simulink model "ANFIS"  (R2015a)
settings: Solver=ode45  StartTime=0.02  StopTime=0.04  RelTol=1e-3
libraries: simulink x36, powerlib_meascontrol x30, powerlib x19, fuzblock x8
(part 1 of 2)
settings Model: Creator=Yahya  LastModifiedBy=Yahya

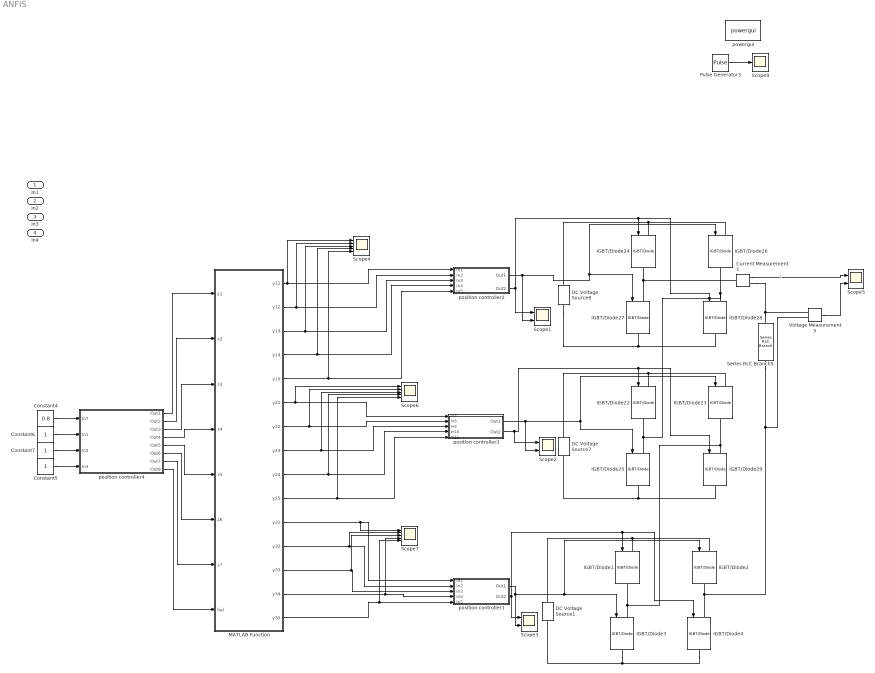
== system ANFIS ==
  note: i
  In1 : Inport
  In2 : Inport  Port=2
  In3 : Inport  Port=3
  In4 : Inport  Port=4
  Constant4 : Constant  Value=0.8
  Constant5 : Constant
  Constant6 : Constant
  Constant7 : Constant
  Current Measurement1 : powerlib/Measurements/Current Measurement  PhasorSimulation=off  OutputType=Complex  PSBequivalent=0
  DC Voltage Source1 : powerlib/Electrical Sources/DC Voltage Source  Amplitude=100  Measurements=None
  DC Voltage Source7 : powerlib/Electrical Sources/DC Voltage Source  Amplitude=100  Measurements=None
  DC Voltage Source8 : powerlib/Electrical Sources/DC Voltage Source  Amplitude=100  Measurements=None
  IGBT/Diode{1..4,22..29} (12 alike) : powerlib/Power Electronics/IGBT//Diode  Ron=1e-3  Rs=1e5  Cs=inf  Measurements=off
  MATLAB Function : MATLAB Function  TreatAsAtomicUnit=on
  Pulse Generator3 : DiscretePulseGenerator  PulseType=Time based  Amplitude=0.8  Period=0.00001  PulseWidth=50
  Scope{1..3,5} (4 alike) : Scope  NumInputPorts=2
      Scope1 settings: TimeRange=1  YMin=-400~-400  YMax=400~400  SaveName=ScopeData7
      Scope2 settings: TimeRange=1  YMin=-400~-400  YMax=400~400  SaveName=ScopeData8
      Scope3 settings: TimeRange=1  YMin=-400~-400  YMax=400~400  SaveName=ScopeData9
      Scope5 settings: TimeRange=1  YMin=-400~-400  YMax=400~400  SaveName=ScopeData3
  Scope4 : Scope  NumInputPorts=5
      settings: TimeRange=1  YMin=-400~-400~-5~-5~-5  YMax=400~400~5~5~5  SaveName=ScopeData12
  Scope6 : Scope  NumInputPorts=5
      settings: TimeRange=1  YMin=-400~-400~-5~-5~-5  YMax=400~400~5~5~5  SaveName=ScopeData13
  Scope7 : Scope  NumInputPorts=5
      settings: TimeRange=1  YMin=-400~-400~-5~-5~-5  YMax=400~400~5~5~5  SaveName=ScopeData14
  Scope9 : Scope
      settings: SaveName=ScopeData18
  Series RLC Branch5 : powerlib/Elements/Series RLC Branch  LConnTagsString=__new0  RConnTagsString=__new0  BranchType=R  Resistance=3000  Inductance=1e-5  SetiL0=off  InitialCurrent=0  Capacitance=1e-6  Setx0=off  InitialVoltage=0  Measurements=None
  Voltage Measurement5 : powerlib/Measurements/Voltage Measurement  PhasorSimulation=off  OutputType=Complex  PSBequivalent=0
  position controller1 : Subsystem
  position controller2 : Subsystem
  position controller3 : Subsystem
  position controller4 : Subsystem
  powergui : powerlib/powergui  Priority=1  SimulationMode=Continuous  SolverType=Tustin/Backward Euler (TBE)  SampleTime=50e-6  frequency=60  SPID=off  DisableSnubberDevices=off  DisableRonSwitches=off  DisableVfSwitches=off  SwTol=0  DisplayEquations=off  Interpol=off  methode=off  Ts=100  FunctionMessages=off  echomessages=off  HookPort=off  EnableUseOfTLC=off  x0status=blocks  frequencyindice=0  Pbase=100e6  ErrMax=1e-4  Iterations=50  UnitsV=kV  UnitsW=MW  buscounter=0  RestoreLinks=warning  ResistiveCurrentMeasurement=off  Frange=[0:2:500]  Ylog=off  Xlog=on  ShowGrid=off  save=off  variable=ZData  structure=0  ZoomFFT=off  StartTime=0.0  cycles=1  DisplayStyle=1  fundamental=60  FreqAxis=off  MaxFrequency=1000  frequencyindicesteady=1  RmsSteady=1  display=off
  wires:
  position controller2/2(Out2) -> Scope1/1, IGBT/Diode28/1, IGBT/Diode24/1
  position controller2/1(Out1) -> Scope1/2, IGBT/Diode26/1, IGBT/Diode27/1
  position controller3/2(Out2) -> Scope2/1, IGBT/Diode29/1, IGBT/Diode22/1
  Current Measurement1/1 -> Scope5/1
  position controller1/2(Out2) -> IGBT/Diode4/1, IGBT/Diode1/1, Scope3/1
  position controller1/1(Out1) -> Scope3/2, IGBT/Diode3/1, IGBT/Diode2/1
  Voltage Measurement5/1 -> Scope5/2
  Pulse Generator3/1 -> Scope9/1
  position controller3/1(Out1) -> Scope2/2, IGBT/Diode23/1, IGBT/Diode25/1
  position controller4/1(Out1) -> MATLAB Function/1(z1)
  position controller4/2(Out2) -> MATLAB Function/2(z2)
  position controller4/3(Out3) -> MATLAB Function/3(z3)
  position controller4/4(Out4) -> MATLAB Function/4(z4)
  position controller4/5(Out5) -> MATLAB Function/5(z5)
  position controller4/6(Out6) -> MATLAB Function/6(z6)
  position controller4/7(Out7) -> MATLAB Function/7(z7)
  position controller4/8(Out8) -> MATLAB Function/8(hal)
  MATLAB Function/1(y11) -> Scope4/1, position controller2/1(In1)
  MATLAB Function/2(y12) -> Scope4/2, position controller2/2(In2)
  MATLAB Function/3(y13) -> Scope4/3, position controller2/3(In3)
  MATLAB Function/4(y14) -> Scope4/4, position controller2/4(In4)
  MATLAB Function/5(y15) -> Scope4/5, position controller2/5(In5)
  MATLAB Function/6(y21) -> Scope6/1, position controller3/1(In7)
  MATLAB Function/7(y22) -> Scope6/2, position controller3/2(In8)
  MATLAB Function/8(y23) -> Scope6/3, position controller3/3(In9)
  MATLAB Function/10(y25) -> Scope6/5, position controller3/5(In11)
  MATLAB Function/11(y31) -> Scope7/1, position controller1/1(In1)
  MATLAB Function/12(y32) -> Scope7/2, position controller1/2(In2)
  MATLAB Function/13(y33) -> Scope7/3, position controller1/3(In3)
  MATLAB Function/14(y34) -> Scope7/4, position controller1/4(In4)
  MATLAB Function/15(y35) -> Scope7/5, position controller1/5(In5)
  Constant4/1 -> position controller4/1(In7)
  Constant6/1 -> position controller4/2(In1)
  Constant7/1 -> position controller4/3(In2)
  Constant5/1 -> position controller4/4(In3)
  MATLAB Function/9(y24) -> Scope6/4, position controller3/4(In10)
  connections:
  IGBT/Diode26/LConn1 -- IGBT/Diode24/LConn1 -- DC Voltage Source8/RConn1
  DC Voltage Source8/LConn1 -- IGBT/Diode28/RConn1 -- IGBT/Diode27/RConn1
  IGBT/Diode27/LConn1 -- Current Measurement1/LConn1 -- IGBT/Diode24/RConn1
  IGBT/Diode23/LConn1 -- IGBT/Diode22/LConn1 -- DC Voltage Source7/RConn1
  IGBT/Diode29/RConn1 -- IGBT/Diode25/RConn1 -- DC Voltage Source7/LConn1
  IGBT/Diode25/LConn1 -- IGBT/Diode26/RConn1 -- IGBT/Diode28/LConn1 -- IGBT/Diode22/RConn1
  IGBT/Diode23/RConn1 -- IGBT/Diode29/LConn1 -- IGBT/Diode1/RConn1 -- IGBT/Diode3/LConn1
  Series RLC Branch5/LConn1 -- Current Measurement1/RConn1 -- Voltage Measurement5/LConn1
  DC Voltage Source1/RConn1 -- IGBT/Diode2/LConn1 -- IGBT/Diode1/LConn1
  DC Voltage Source1/LConn1 -- IGBT/Diode4/RConn1 -- IGBT/Diode3/RConn1
  Voltage Measurement5/LConn2 -- Series RLC Branch5/RConn1 -- IGBT/Diode4/LConn1 -- IGBT/Diode2/RConn1

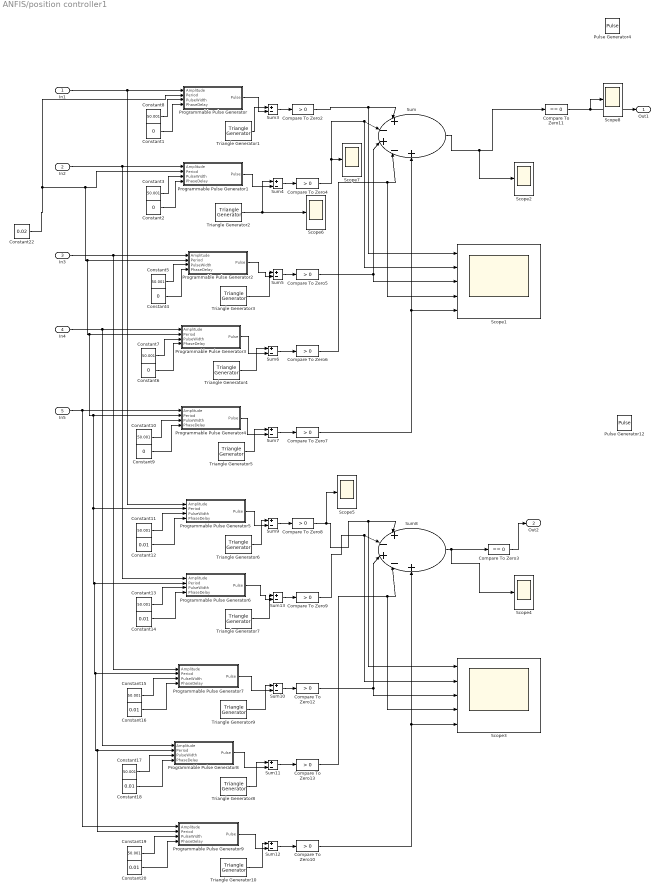
== system ANFIS/position controller1 ==
  In1 : Inport
  In2 : Inport  Port=2
  In3 : Inport  Port=3
  In4 : Inport  Port=4
  In5 : Inport  Port=5
  Compare To Zero{2,4..10,12..13} (10 alike) : simulink/Logic and Bit Operations/Compare To Zero  relop=>  OutDataTypeStr=boolean  ZeroCross=off
  Compare To Zero11 : simulink/Logic and Bit Operations/Compare To Zero  relop===  OutDataTypeStr=boolean  ZeroCross=off
  Compare To Zero3 : simulink/Logic and Bit Operations/Compare To Zero  relop===  OutDataTypeStr=boolean  ZeroCross=off
  Constant{1..2,4,6,9} (5 alike) : Constant  Value=0
  Constant{3,5,7..8,10..11,13,15,17,19} (10 alike) : Constant  Value=50.001
  Constant{12,14,16,18,20} (5 alike) : Constant  Value=0.01
  Constant22 : Constant  Value=0.02
  Programmable Pulse Generator : Subsystem
  Programmable Pulse Generator1 : Subsystem
  Programmable Pulse Generator2 : Subsystem
  Programmable Pulse Generator3 : Subsystem
  Programmable Pulse Generator4 : Subsystem
  Programmable Pulse Generator5 : Subsystem
  Programmable Pulse Generator6 : Subsystem
  Programmable Pulse Generator7 : Subsystem
  Programmable Pulse Generator8 : Subsystem
  Programmable Pulse Generator9 : Subsystem
  Pulse Generator12 : DiscretePulseGenerator  PulseType=Time based  Amplitude=0.289737494146879  Period=0.02  PulseWidth=50.001  PhaseDelay=0.01
  Pulse Generator4 : DiscretePulseGenerator  PulseType=Time based  Amplitude=0.289737494146879  Period=0.02  PulseWidth=50.001
  Scope1 : Scope  NumInputPorts=5
      settings: TimeRange=0.02  YMin=0~0~0~0~0  YMax=1~1~1~1~1
  Scope{2,4..8} (6 alike) : Scope
      Scope4 settings: SaveName=ScopeData4
      Scope5 settings: SaveName=ScopeData5
      Scope6 settings: SaveName=ScopeData6
      Scope7 settings: SaveName=ScopeData10
      Scope8 settings: SaveName=ScopeData11
  Scope3 : Scope  NumInputPorts=5
      settings: YMin=-5~-5~-5~-5~-5  YMax=5~5~5~5~5  SaveName=ScopeData2
  Sum : Sum  Inputs=|+-+-+
  Sum{3..7,9..13} (10 alike) : Sum  Inputs=+-  OutDataTypeStr=double
  Sum8 : Sum  Inputs=|+-+-+
  Triangle Generator{1..5} (5 alike) : powerlib_meascontrol/Pulse & Signal Generators/Triangle Generator  Freq=50  Phase=90  Ts=0
  Triangle Generator{6..10} (5 alike) : powerlib_meascontrol/Pulse & Signal Generators/Triangle Generator  Freq=50  Phase=90+180  Ts=0
  Out1 : Outport
  Out2 : Outport  Port=2
  wires:
  Triangle Generator1/1 -> Sum3/1
  Sum3/1 -> Compare To Zero2/1
  Programmable Pulse Generator/1(Pulse) -> Sum3/2
  Triangle Generator2/1 -> Sum4/1, Scope6/1
  Sum4/1 -> Compare To Zero4/1
  Programmable Pulse Generator1/1(Pulse) -> Sum4/2
  Triangle Generator3/1 -> Sum5/1
  Sum5/1 -> Compare To Zero5/1
  Programmable Pulse Generator2/1(Pulse) -> Sum5/2
  Triangle Generator4/1 -> Sum6/1
  Sum6/1 -> Compare To Zero6/1
  Programmable Pulse Generator3/1(Pulse) -> Sum6/2
  Triangle Generator5/1 -> Sum7/1
  Sum7/1 -> Compare To Zero7/1
  Programmable Pulse Generator4/1(Pulse) -> Sum7/2
  Compare To Zero2/1 -> Scope1/1, Sum/1
  Compare To Zero5/1 -> Sum/3, Scope1/3
  Sum/1 -> Scope2/1, Compare To Zero11/1
  Compare To Zero6/1 -> Scope1/4, Sum/4
  Compare To Zero7/1 -> Scope1/5, Sum/5
  Triangle Generator6/1 -> Sum9/1
  Sum9/1 -> Compare To Zero8/1
  Programmable Pulse Generator5/1(Pulse) -> Sum9/2
  Triangle Generator7/1 -> Sum13/1
  Sum13/1 -> Compare To Zero9/1
  Programmable Pulse Generator6/1(Pulse) -> Sum13/2
  Triangle Generator9/1 -> Sum10/1
  Sum10/1 -> Compare To Zero12/1
  Programmable Pulse Generator7/1(Pulse) -> Sum10/2
  Triangle Generator8/1 -> Sum11/1
  Sum11/1 -> Compare To Zero13/1
  Programmable Pulse Generator8/1(Pulse) -> Sum11/2
  Triangle Generator10/1 -> Sum12/1
  Sum12/1 -> Compare To Zero10/1
  Programmable Pulse Generator9/1(Pulse) -> Sum12/2
  Compare To Zero8/1 -> Scope5/1, Scope3/1, Sum8/1
  Compare To Zero9/1 -> Scope3/2, Sum8/2
  Compare To Zero12/1 -> Sum8/3, Scope3/3
  Sum8/1 -> Scope4/1, Compare To Zero3/1
  Compare To Zero13/1 -> Scope3/4, Sum8/4
  Compare To Zero10/1 -> Scope3/5, Sum8/5
  Compare To Zero4/1 -> Scope1/2, Sum/2, Scope7/1
  Compare To Zero11/1 -> Scope8/1, Out1/1
  Compare To Zero3/1 -> Out2/1
  Constant8/1 -> Programmable Pulse Generator/3(PulseWidth)
  Constant1/1 -> Programmable Pulse Generator/4(PhaseDelay)
  Constant3/1 -> Programmable Pulse Generator1/3(PulseWidth)
  Constant2/1 -> Programmable Pulse Generator1/4(PhaseDelay)
  Constant4/1 -> Programmable Pulse Generator2/4(PhaseDelay)
  Constant5/1 -> Programmable Pulse Generator2/3(PulseWidth)
  Constant6/1 -> Programmable Pulse Generator3/4(PhaseDelay)
  Constant7/1 -> Programmable Pulse Generator3/3(PulseWidth)
  Constant9/1 -> Programmable Pulse Generator4/4(PhaseDelay)
  Constant10/1 -> Programmable Pulse Generator4/3(PulseWidth)
  Constant12/1 -> Programmable Pulse Generator5/4(PhaseDelay)
  Constant11/1 -> Programmable Pulse Generator5/3(PulseWidth)
  Constant14/1 -> Programmable Pulse Generator6/4(PhaseDelay)
  Constant13/1 -> Programmable Pulse Generator6/3(PulseWidth)
  Constant16/1 -> Programmable Pulse Generator7/4(PhaseDelay)
  Constant15/1 -> Programmable Pulse Generator7/3(PulseWidth)
  Constant18/1 -> Programmable Pulse Generator8/4(PhaseDelay)
  Constant17/1 -> Programmable Pulse Generator8/3(PulseWidth)
  Constant20/1 -> Programmable Pulse Generator9/4(PhaseDelay)
  Constant19/1 -> Programmable Pulse Generator9/3(PulseWidth)
  In1/1 -> Programmable Pulse Generator5/1(Amplitude), Programmable Pulse Generator/1(Amplitude)
  In2/1 -> Programmable Pulse Generator6/1(Amplitude), Programmable Pulse Generator1/1(Amplitude)
  In3/1 -> Programmable Pulse Generator7/1(Amplitude), Programmable Pulse Generator2/1(Amplitude)
  In4/1 -> Programmable Pulse Generator8/1(Amplitude), Programmable Pulse Generator3/1(Amplitude)
  In5/1 -> Programmable Pulse Generator9/1(Amplitude), Programmable Pulse Generator4/1(Amplitude)
  Constant22/1 -> Programmable Pulse Generator9/2(Period), Programmable Pulse Generator8/2(Period), Programmable Pulse Generator7/2(Period), Programmable Pulse Generator6/2(Period), Programmable Pulse Generator5/2(Period), Programmable Pulse Generator4/2(Period), Programmable Pulse Generator3/2(Period), Programmable Pulse Generator2/2(Period), Programmable Pulse Generator1/2(Period), Programmable Pulse Generator/2(Period)

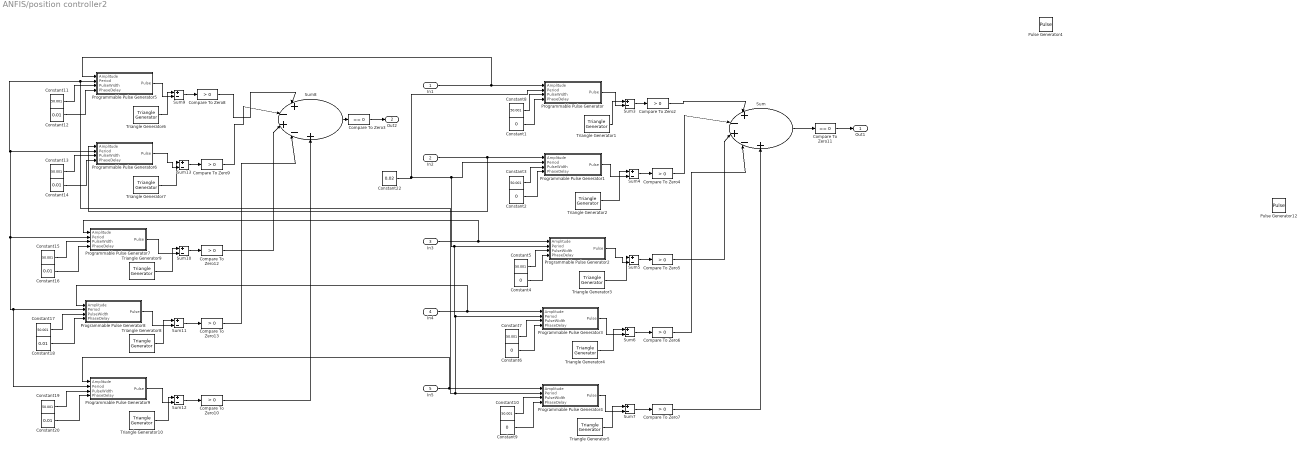
== system ANFIS/position controller2 ==
  In1 : Inport
  In2 : Inport  Port=2
  In3 : Inport  Port=3
  In4 : Inport  Port=4
  In5 : Inport  Port=5
  Compare To Zero{2,4..10,12..13} (10 alike) : simulink/Logic and Bit Operations/Compare To Zero  relop=>  OutDataTypeStr=boolean  ZeroCross=off
  Compare To Zero11 : simulink/Logic and Bit Operations/Compare To Zero  relop===  OutDataTypeStr=boolean  ZeroCross=off
  Compare To Zero3 : simulink/Logic and Bit Operations/Compare To Zero  relop===  OutDataTypeStr=boolean  ZeroCross=off
  Constant{1..2,4,6,9} (5 alike) : Constant  Value=0
  Constant{3,5,7..8,10..11,13,15,17,19} (10 alike) : Constant  Value=50.001
  Constant{12,14,16,18,20} (5 alike) : Constant  Value=0.01
  Constant22 : Constant  Value=0.02
  Programmable Pulse Generator : Subsystem
  Programmable Pulse Generator1 : Subsystem
  Programmable Pulse Generator2 : Subsystem
  Programmable Pulse Generator3 : Subsystem
  Programmable Pulse Generator4 : Subsystem
  Programmable Pulse Generator5 : Subsystem
  Programmable Pulse Generator6 : Subsystem
  Programmable Pulse Generator7 : Subsystem
  Programmable Pulse Generator8 : Subsystem
  Programmable Pulse Generator9 : Subsystem
  Pulse Generator12 : DiscretePulseGenerator  PulseType=Time based  Amplitude=0.289737494146879  Period=0.02  PulseWidth=50.001  PhaseDelay=0.01
  Pulse Generator4 : DiscretePulseGenerator  PulseType=Time based  Amplitude=0.289737494146879  Period=0.02  PulseWidth=50.001
  Sum : Sum  Inputs=|+-+-+
  Sum{3..7,9..13} (10 alike) : Sum  Inputs=+-  OutDataTypeStr=double
  Sum8 : Sum  Inputs=|+-+-+
  Triangle Generator{1..5} (5 alike) : powerlib_meascontrol/Pulse & Signal Generators/Triangle Generator  Freq=50  Phase=90  Ts=0
  Triangle Generator{6..10} (5 alike) : powerlib_meascontrol/Pulse & Signal Generators/Triangle Generator  Freq=50  Phase=90+180  Ts=0
  Out1 : Outport
  Out2 : Outport  Port=2
  wires:
  Triangle Generator1/1 -> Sum3/1
  Sum3/1 -> Compare To Zero2/1
  Programmable Pulse Generator/1(Pulse) -> Sum3/2
  Triangle Generator2/1 -> Sum4/1
  Sum4/1 -> Compare To Zero4/1
  Programmable Pulse Generator1/1(Pulse) -> Sum4/2
  Triangle Generator3/1 -> Sum5/1
  Sum5/1 -> Compare To Zero5/1
  Programmable Pulse Generator2/1(Pulse) -> Sum5/2
  Triangle Generator4/1 -> Sum6/1
  Sum6/1 -> Compare To Zero6/1
  Programmable Pulse Generator3/1(Pulse) -> Sum6/2
  Triangle Generator5/1 -> Sum7/1
  Sum7/1 -> Compare To Zero7/1
  Programmable Pulse Generator4/1(Pulse) -> Sum7/2
  Compare To Zero2/1 -> Sum/1
  Compare To Zero5/1 -> Sum/3
  Sum/1 -> Compare To Zero11/1
  Compare To Zero6/1 -> Sum/4
  Compare To Zero7/1 -> Sum/5
  Triangle Generator6/1 -> Sum9/1
  Sum9/1 -> Compare To Zero8/1
  Programmable Pulse Generator5/1(Pulse) -> Sum9/2
  Triangle Generator7/1 -> Sum13/1
  Sum13/1 -> Compare To Zero9/1
  Programmable Pulse Generator6/1(Pulse) -> Sum13/2
  Triangle Generator9/1 -> Sum10/1
  Sum10/1 -> Compare To Zero12/1
  Programmable Pulse Generator7/1(Pulse) -> Sum10/2
  Triangle Generator8/1 -> Sum11/1
  Sum11/1 -> Compare To Zero13/1
  Programmable Pulse Generator8/1(Pulse) -> Sum11/2
  Triangle Generator10/1 -> Sum12/1
  Sum12/1 -> Compare To Zero10/1
  Programmable Pulse Generator9/1(Pulse) -> Sum12/2
  Compare To Zero8/1 -> Sum8/1
  Compare To Zero9/1 -> Sum8/2
  Compare To Zero12/1 -> Sum8/3
  Sum8/1 -> Compare To Zero3/1
  Compare To Zero13/1 -> Sum8/4
  Compare To Zero10/1 -> Sum8/5
  Compare To Zero4/1 -> Sum/2
  Compare To Zero11/1 -> Out1/1
  Compare To Zero3/1 -> Out2/1
  Constant8/1 -> Programmable Pulse Generator/3(PulseWidth)
  Constant1/1 -> Programmable Pulse Generator/4(PhaseDelay)
  Constant3/1 -> Programmable Pulse Generator1/3(PulseWidth)
  Constant2/1 -> Programmable Pulse Generator1/4(PhaseDelay)
  Constant4/1 -> Programmable Pulse Generator2/4(PhaseDelay)
  Constant5/1 -> Programmable Pulse Generator2/3(PulseWidth)
  Constant6/1 -> Programmable Pulse Generator3/4(PhaseDelay)
  Constant7/1 -> Programmable Pulse Generator3/3(PulseWidth)
  Constant9/1 -> Programmable Pulse Generator4/4(PhaseDelay)
  Constant10/1 -> Programmable Pulse Generator4/3(PulseWidth)
  Constant12/1 -> Programmable Pulse Generator5/4(PhaseDelay)
  Constant11/1 -> Programmable Pulse Generator5/3(PulseWidth)
  Constant14/1 -> Programmable Pulse Generator6/4(PhaseDelay)
  Constant13/1 -> Programmable Pulse Generator6/3(PulseWidth)
  Constant16/1 -> Programmable Pulse Generator7/4(PhaseDelay)
  Constant15/1 -> Programmable Pulse Generator7/3(PulseWidth)
  Constant18/1 -> Programmable Pulse Generator8/4(PhaseDelay)
  Constant17/1 -> Programmable Pulse Generator8/3(PulseWidth)
  Constant20/1 -> Programmable Pulse Generator9/4(PhaseDelay)
  Constant19/1 -> Programmable Pulse Generator9/3(PulseWidth)
  In1/1 -> Programmable Pulse Generator5/1(Amplitude), Programmable Pulse Generator/1(Amplitude)
  In2/1 -> Programmable Pulse Generator6/1(Amplitude), Programmable Pulse Generator1/1(Amplitude)
  In3/1 -> Programmable Pulse Generator7/1(Amplitude), Programmable Pulse Generator2/1(Amplitude)
  In4/1 -> Programmable Pulse Generator8/1(Amplitude), Programmable Pulse Generator3/1(Amplitude)
  In5/1 -> Programmable Pulse Generator9/1(Amplitude), Programmable Pulse Generator4/1(Amplitude)
  Constant22/1 -> Programmable Pulse Generator4/2(Period), Programmable Pulse Generator5/2(Period), Programmable Pulse Generator9/2(Period), Programmable Pulse Generator8/2(Period), Programmable Pulse Generator7/2(Period), Programmable Pulse Generator6/2(Period), Programmable Pulse Generator3/2(Period), Programmable Pulse Generator2/2(Period), Programmable Pulse Generator1/2(Period), Programmable Pulse Generator/2(Period)

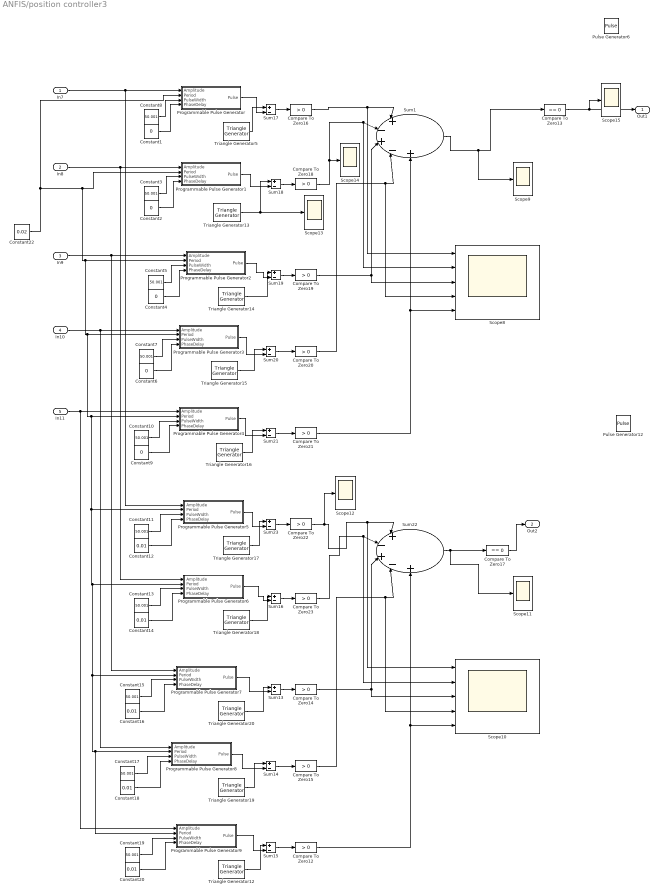
== system ANFIS/position controller3 ==
  In7 : Inport
  In8 : Inport  Port=2
  In9 : Inport  Port=3
  In10 : Inport  Port=4
  In11 : Inport  Port=5
  Compare To Zero{12,14..16,18..23} (10 alike) : simulink/Logic and Bit Operations/Compare To Zero  relop=>  OutDataTypeStr=boolean  ZeroCross=off
  Compare To Zero13 : simulink/Logic and Bit Operations/Compare To Zero  relop===  OutDataTypeStr=boolean  ZeroCross=off
  Compare To Zero17 : simulink/Logic and Bit Operations/Compare To Zero  relop===  OutDataTypeStr=boolean  ZeroCross=off
  Constant{1..2,4,6,9} (5 alike) : Constant  Value=0
  Constant{3,5,7..8,10..11,13,15,17,19} (10 alike) : Constant  Value=50.001
  Constant{12,14,16,18,20} (5 alike) : Constant  Value=0.01
  Constant22 : Constant  Value=0.02
  Programmable Pulse Generator : Subsystem
  Programmable Pulse Generator1 : Subsystem
  Programmable Pulse Generator2 : Subsystem
  Programmable Pulse Generator3 : Subsystem
  Programmable Pulse Generator4 : Subsystem
  Programmable Pulse Generator5 : Subsystem
  Programmable Pulse Generator6 : Subsystem
  Programmable Pulse Generator7 : Subsystem
  Programmable Pulse Generator8 : Subsystem
  Programmable Pulse Generator9 : Subsystem
  Pulse Generator12 : DiscretePulseGenerator  PulseType=Time based  Amplitude=0.289737494146879  Period=0.02  PulseWidth=50.001  PhaseDelay=0.01
  Pulse Generator6 : DiscretePulseGenerator  PulseType=Time based  Amplitude=0.289737494146879  Period=0.02  PulseWidth=50.001
  Scope10 : Scope  NumInputPorts=5
      settings: YMin=-5~-5~-5~-5~-5  YMax=5~5~5~5~5  SaveName=ScopeData28
  Scope{9,11..15} (6 alike) : Scope
      Scope11 settings: SaveName=ScopeData29
      Scope12 settings: SaveName=ScopeData30
      Scope13 settings: SaveName=ScopeData31
      Scope14 settings: SaveName=ScopeData32
      Scope15 settings: SaveName=ScopeData33
      Scope9 settings: SaveName=ScopeData35
  Scope8 : Scope  NumInputPorts=5
      settings: TimeRange=0.02  YMin=0~0~0~0~0  YMax=1~1~1~1~1  SaveName=ScopeData34
  Sum1 : Sum  Inputs=|+-+-+
  Sum{13..21,23} (10 alike) : Sum  Inputs=+-  OutDataTypeStr=double
  Sum22 : Sum  Inputs=|+-+-+
  Triangle Generator{12,17..20} (5 alike) : powerlib_meascontrol/Pulse & Signal Generators/Triangle Generator  Freq=50  Phase=90+180  Ts=0
  Triangle Generator{5,13..16} (5 alike) : powerlib_meascontrol/Pulse & Signal Generators/Triangle Generator  Freq=50  Phase=90  Ts=0
  Out1 : Outport
  Out2 : Outport  Port=2
  wires:
  Triangle Generator5/1 -> Sum17/1
  Sum17/1 -> Compare To Zero16/1
  Programmable Pulse Generator/1(Pulse) -> Sum17/2
  Triangle Generator13/1 -> Sum18/1, Scope13/1
  Sum18/1 -> Compare To Zero18/1
  Programmable Pulse Generator1/1(Pulse) -> Sum18/2
  Triangle Generator14/1 -> Sum19/1
  Sum19/1 -> Compare To Zero19/1
  Programmable Pulse Generator2/1(Pulse) -> Sum19/2
  Triangle Generator15/1 -> Sum20/1
  Sum20/1 -> Compare To Zero20/1
  Programmable Pulse Generator3/1(Pulse) -> Sum20/2
  Triangle Generator16/1 -> Sum21/1
  Sum21/1 -> Compare To Zero21/1
  Programmable Pulse Generator4/1(Pulse) -> Sum21/2
  Compare To Zero16/1 -> Scope8/1, Sum1/1
  Compare To Zero19/1 -> Sum1/3, Scope8/3
  Sum1/1 -> Scope9/1, Compare To Zero13/1
  Compare To Zero20/1 -> Scope8/4, Sum1/4
  Compare To Zero21/1 -> Scope8/5, Sum1/5
  Triangle Generator17/1 -> Sum23/1
  Sum23/1 -> Compare To Zero22/1
  Programmable Pulse Generator5/1(Pulse) -> Sum23/2
  Triangle Generator18/1 -> Sum16/1
  Sum16/1 -> Compare To Zero23/1
  Programmable Pulse Generator6/1(Pulse) -> Sum16/2
  Triangle Generator20/1 -> Sum13/1
  Sum13/1 -> Compare To Zero14/1
  Programmable Pulse Generator7/1(Pulse) -> Sum13/2
  Triangle Generator19/1 -> Sum14/1
  Sum14/1 -> Compare To Zero15/1
  Programmable Pulse Generator8/1(Pulse) -> Sum14/2
  Triangle Generator12/1 -> Sum15/1
  Sum15/1 -> Compare To Zero12/1
  Programmable Pulse Generator9/1(Pulse) -> Sum15/2
  Compare To Zero22/1 -> Scope12/1, Scope10/1, Sum22/1
  Compare To Zero23/1 -> Scope10/2, Sum22/2
  Compare To Zero14/1 -> Sum22/3, Scope10/3
  Sum22/1 -> Scope11/1, Compare To Zero17/1
  Compare To Zero15/1 -> Scope10/4, Sum22/4
  Compare To Zero12/1 -> Scope10/5, Sum22/5
  Compare To Zero18/1 -> Scope8/2, Sum1/2, Scope14/1
  Compare To Zero13/1 -> Scope15/1, Out1/1
  Compare To Zero17/1 -> Out2/1
  Constant8/1 -> Programmable Pulse Generator/3(PulseWidth)
  Constant1/1 -> Programmable Pulse Generator/4(PhaseDelay)
  Constant3/1 -> Programmable Pulse Generator1/3(PulseWidth)
  Constant2/1 -> Programmable Pulse Generator1/4(PhaseDelay)
  Constant4/1 -> Programmable Pulse Generator2/4(PhaseDelay)
  Constant5/1 -> Programmable Pulse Generator2/3(PulseWidth)
  Constant6/1 -> Programmable Pulse Generator3/4(PhaseDelay)
  Constant7/1 -> Programmable Pulse Generator3/3(PulseWidth)
  Constant9/1 -> Programmable Pulse Generator4/4(PhaseDelay)
  Constant10/1 -> Programmable Pulse Generator4/3(PulseWidth)
  Constant12/1 -> Programmable Pulse Generator5/4(PhaseDelay)
  Constant11/1 -> Programmable Pulse Generator5/3(PulseWidth)
  Constant14/1 -> Programmable Pulse Generator6/4(PhaseDelay)
  Constant13/1 -> Programmable Pulse Generator6/3(PulseWidth)
  Constant16/1 -> Programmable Pulse Generator7/4(PhaseDelay)
  Constant15/1 -> Programmable Pulse Generator7/3(PulseWidth)
  Constant18/1 -> Programmable Pulse Generator8/4(PhaseDelay)
  Constant17/1 -> Programmable Pulse Generator8/3(PulseWidth)
  Constant20/1 -> Programmable Pulse Generator9/4(PhaseDelay)
  Constant19/1 -> Programmable Pulse Generator9/3(PulseWidth)
  In7/1 -> Programmable Pulse Generator5/1(Amplitude), Programmable Pulse Generator/1(Amplitude)
  In8/1 -> Programmable Pulse Generator6/1(Amplitude), Programmable Pulse Generator1/1(Amplitude)
  In9/1 -> Programmable Pulse Generator7/1(Amplitude), Programmable Pulse Generator2/1(Amplitude)
  In10/1 -> Programmable Pulse Generator8/1(Amplitude), Programmable Pulse Generator3/1(Amplitude)
  In11/1 -> Programmable Pulse Generator9/1(Amplitude), Programmable Pulse Generator4/1(Amplitude)
  Constant22/1 -> Programmable Pulse Generator9/2(Period), Programmable Pulse Generator8/2(Period), Programmable Pulse Generator7/2(Period), Programmable Pulse Generator6/2(Period), Programmable Pulse Generator5/2(Period), Programmable Pulse Generator4/2(Period), Programmable Pulse Generator3/2(Period), Programmable Pulse Generator2/2(Period), Programmable Pulse Generator1/2(Period), Programmable Pulse Generator/2(Period)

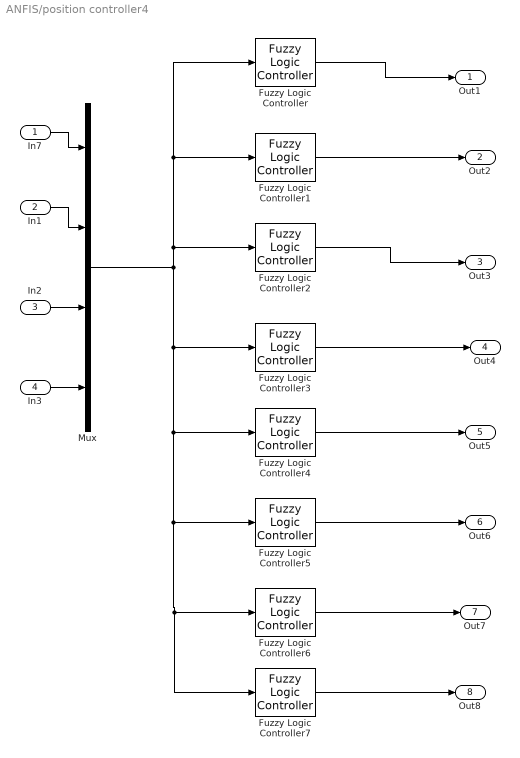
== system ANFIS/position controller4 ==
  In7 : Inport
  In1 : Inport  Port=2
  In2 : Inport  Port=3
  In3 : Inport  Port=4
  Fuzzy Logic Controller : fuzblock/Fuzzy Logic  Controller  fis='ANFIS_1_F.fis'
  Fuzzy Logic Controller1 : fuzblock/Fuzzy Logic  Controller  fis='ANFIS_2_F.fis'
  Fuzzy Logic Controller2 : fuzblock/Fuzzy Logic  Controller  fis='ANFIS_3_F.fis'
  Fuzzy Logic Controller3 : fuzblock/Fuzzy Logic  Controller  fis='ANFIS_4_F.fis'
  Fuzzy Logic Controller4 : fuzblock/Fuzzy Logic  Controller  fis='ANFIS_5_F.fis'
  Fuzzy Logic Controller5 : fuzblock/Fuzzy Logic  Controller  fis='ANFIS_6_F.fis'
  Fuzzy Logic Controller6 : fuzblock/Fuzzy Logic  Controller  fis='ANFIS_7_F.fis'
  Fuzzy Logic Controller7 : fuzblock/Fuzzy Logic  Controller  fis='ANFIS_8_F.fis'
  Mux : Mux
  Out1 : Outport
  Out2 : Outport  Port=2
  Out3 : Outport  Port=3
  Out4 : Outport  Port=4
  Out5 : Outport  Port=5
  Out6 : Outport  Port=6
  Out7 : Outport  Port=7
  Out8 : Outport  Port=8
  wires:
  In7/1 -> Mux/1
  In1/1 -> Mux/2
  In2/1 -> Mux/3
  In3/1 -> Mux/4
  Mux/1 -> Fuzzy Logic Controller2/1, Fuzzy Logic Controller1/1, Fuzzy Logic Controller/1, Fuzzy Logic Controller3/1, Fuzzy Logic Controller4/1, Fuzzy Logic Controller5/1, Fuzzy Logic Controller7/1, Fuzzy Logic Controller6/1
  Fuzzy Logic Controller/1 -> Out1/1
  Fuzzy Logic Controller1/1 -> Out2/1
  Fuzzy Logic Controller2/1 -> Out3/1
  Fuzzy Logic Controller3/1 -> Out4/1
  Fuzzy Logic Controller4/1 -> Out5/1
  Fuzzy Logic Controller5/1 -> Out6/1
  Fuzzy Logic Controller6/1 -> Out7/1
  Fuzzy Logic Controller7/1 -> Out8/1

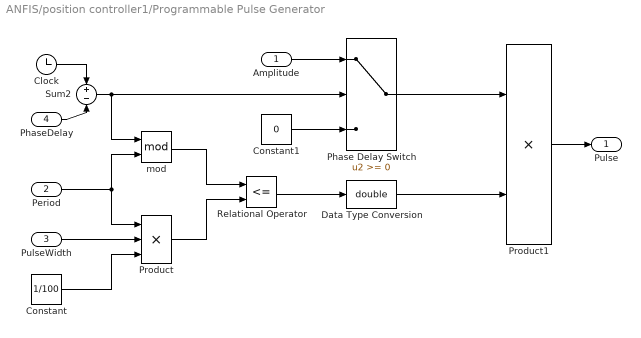
== system ANFIS/position controller1/Programmable Pulse Generator ==
  Amplitude : Inport
  Period : Inport  Port=2
  PulseWidth : Inport  Port=3
  PhaseDelay : Inport  Port=4
  Clock : Clock
  Constant : Constant  Value=1/100
  Constant1 : Constant  Value=0
  Data Type Conversion : DataTypeConversion  OutDataTypeStr=double
  Phase Delay Switch : Switch
  Product : Product  Inputs=3  RndMeth=Zero
  Product1 : Product  RndMeth=Zero
  Relational Operator : RelationalOperator  Operator=<=
  Sum2 : Sum  Inputs=+-
  mod : Math  Operator=mod  SaturateOnIntegerOverflow=on
  Pulse : Outport
  wires:
  Product/1 -> Relational Operator/2
  Product1/1 -> Pulse/1
  Data Type Conversion/1 -> Product1/2
  Relational Operator/1 -> Data Type Conversion/1
  Constant/1 -> Product/3
  PulseWidth/1 -> Product/2
  mod/1 -> Relational Operator/1
  Period/1 -> Product/1, mod/2
  Clock/1 -> Sum2/1
  PhaseDelay/1 -> Sum2/2
  Sum2/1 -> mod/1, Phase Delay Switch/2
  Amplitude/1 -> Phase Delay Switch/1
  Constant1/1 -> Phase Delay Switch/3
  Phase Delay Switch/1 -> Product1/1

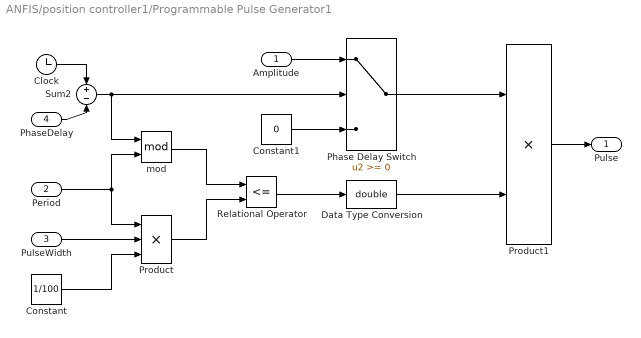
== system ANFIS/position controller1/Programmable Pulse Generator1 ==
  Amplitude : Inport
  Period : Inport  Port=2
  PulseWidth : Inport  Port=3
  PhaseDelay : Inport  Port=4
  Clock : Clock
  Constant : Constant  Value=1/100
  Constant1 : Constant  Value=0
  Data Type Conversion : DataTypeConversion  OutDataTypeStr=double
  Phase Delay Switch : Switch
  Product : Product  Inputs=3  RndMeth=Zero
  Product1 : Product  RndMeth=Zero
  Relational Operator : RelationalOperator  Operator=<=
  Sum2 : Sum  Inputs=+-
  mod : Math  Operator=mod  SaturateOnIntegerOverflow=on
  Pulse : Outport
  wires:
  Phase Delay Switch/1 -> Product1/1
  Constant1/1 -> Phase Delay Switch/3
  Amplitude/1 -> Phase Delay Switch/1
  Sum2/1 -> Phase Delay Switch/2, mod/1
  PhaseDelay/1 -> Sum2/2
  Clock/1 -> Sum2/1
  Period/1 -> mod/2, Product/1
  mod/1 -> Relational Operator/1
  PulseWidth/1 -> Product/2
  Constant/1 -> Product/3
  Relational Operator/1 -> Data Type Conversion/1
  Data Type Conversion/1 -> Product1/2
  Product1/1 -> Pulse/1
  Product/1 -> Relational Operator/2

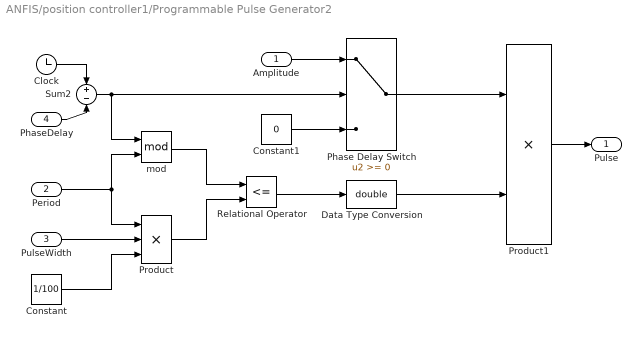
== system ANFIS/position controller1/Programmable Pulse Generator2 ==
  Amplitude : Inport
  Period : Inport  Port=2
  PulseWidth : Inport  Port=3
  PhaseDelay : Inport  Port=4
  Clock : Clock
  Constant : Constant  Value=1/100
  Constant1 : Constant  Value=0
  Data Type Conversion : DataTypeConversion  OutDataTypeStr=double
  Phase Delay Switch : Switch
  Product : Product  Inputs=3  RndMeth=Zero
  Product1 : Product  RndMeth=Zero
  Relational Operator : RelationalOperator  Operator=<=
  Sum2 : Sum  Inputs=+-
  mod : Math  Operator=mod  SaturateOnIntegerOverflow=on
  Pulse : Outport
  wires:
  Product/1 -> Relational Operator/2
  Product1/1 -> Pulse/1
  Data Type Conversion/1 -> Product1/2
  Relational Operator/1 -> Data Type Conversion/1
  Constant/1 -> Product/3
  PulseWidth/1 -> Product/2
  mod/1 -> Relational Operator/1
  Period/1 -> Product/1, mod/2
  Clock/1 -> Sum2/1
  PhaseDelay/1 -> Sum2/2
  Sum2/1 -> mod/1, Phase Delay Switch/2
  Amplitude/1 -> Phase Delay Switch/1
  Constant1/1 -> Phase Delay Switch/3
  Phase Delay Switch/1 -> Product1/1

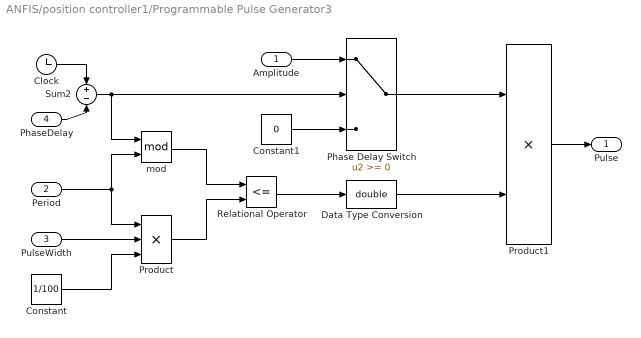
== system ANFIS/position controller1/Programmable Pulse Generator3 ==
  Amplitude : Inport
  Period : Inport  Port=2
  PulseWidth : Inport  Port=3
  PhaseDelay : Inport  Port=4
  Clock : Clock
  Constant : Constant  Value=1/100
  Constant1 : Constant  Value=0
  Data Type Conversion : DataTypeConversion  OutDataTypeStr=double
  Phase Delay Switch : Switch
  Product : Product  Inputs=3  RndMeth=Zero
  Product1 : Product  RndMeth=Zero
  Relational Operator : RelationalOperator  Operator=<=
  Sum2 : Sum  Inputs=+-
  mod : Math  Operator=mod  SaturateOnIntegerOverflow=on
  Pulse : Outport
  wires:
  Phase Delay Switch/1 -> Product1/1
  Constant1/1 -> Phase Delay Switch/3
  Amplitude/1 -> Phase Delay Switch/1
  Sum2/1 -> Phase Delay Switch/2, mod/1
  PhaseDelay/1 -> Sum2/2
  Clock/1 -> Sum2/1
  Period/1 -> mod/2, Product/1
  mod/1 -> Relational Operator/1
  PulseWidth/1 -> Product/2
  Constant/1 -> Product/3
  Relational Operator/1 -> Data Type Conversion/1
  Data Type Conversion/1 -> Product1/2
  Product1/1 -> Pulse/1
  Product/1 -> Relational Operator/2

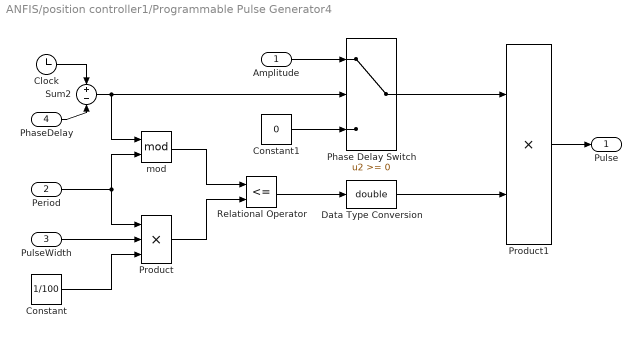
== system ANFIS/position controller1/Programmable Pulse Generator4 ==
  Amplitude : Inport
  Period : Inport  Port=2
  PulseWidth : Inport  Port=3
  PhaseDelay : Inport  Port=4
  Clock : Clock
  Constant : Constant  Value=1/100
  Constant1 : Constant  Value=0
  Data Type Conversion : DataTypeConversion  OutDataTypeStr=double
  Phase Delay Switch : Switch
  Product : Product  Inputs=3  RndMeth=Zero
  Product1 : Product  RndMeth=Zero
  Relational Operator : RelationalOperator  Operator=<=
  Sum2 : Sum  Inputs=+-
  mod : Math  Operator=mod  SaturateOnIntegerOverflow=on
  Pulse : Outport
  wires:
  Product/1 -> Relational Operator/2
  Product1/1 -> Pulse/1
  Data Type Conversion/1 -> Product1/2
  Relational Operator/1 -> Data Type Conversion/1
  Constant/1 -> Product/3
  PulseWidth/1 -> Product/2
  mod/1 -> Relational Operator/1
  Period/1 -> Product/1, mod/2
  Clock/1 -> Sum2/1
  PhaseDelay/1 -> Sum2/2
  Sum2/1 -> mod/1, Phase Delay Switch/2
  Amplitude/1 -> Phase Delay Switch/1
  Constant1/1 -> Phase Delay Switch/3
  Phase Delay Switch/1 -> Product1/1

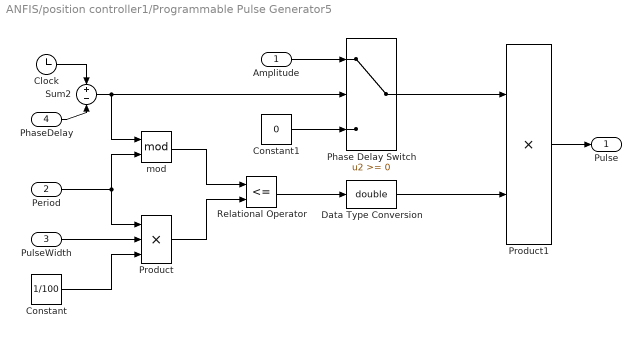
== system ANFIS/position controller1/Programmable Pulse Generator5 ==
  Amplitude : Inport
  Period : Inport  Port=2
  PulseWidth : Inport  Port=3
  PhaseDelay : Inport  Port=4
  Clock : Clock
  Constant : Constant  Value=1/100
  Constant1 : Constant  Value=0
  Data Type Conversion : DataTypeConversion  OutDataTypeStr=double
  Phase Delay Switch : Switch
  Product : Product  Inputs=3  RndMeth=Zero
  Product1 : Product  RndMeth=Zero
  Relational Operator : RelationalOperator  Operator=<=
  Sum2 : Sum  Inputs=+-
  mod : Math  Operator=mod  SaturateOnIntegerOverflow=on
  Pulse : Outport
  wires:
  Phase Delay Switch/1 -> Product1/1
  Constant1/1 -> Phase Delay Switch/3
  Amplitude/1 -> Phase Delay Switch/1
  Sum2/1 -> Phase Delay Switch/2, mod/1
  PhaseDelay/1 -> Sum2/2
  Clock/1 -> Sum2/1
  Period/1 -> mod/2, Product/1
  mod/1 -> Relational Operator/1
  PulseWidth/1 -> Product/2
  Constant/1 -> Product/3
  Relational Operator/1 -> Data Type Conversion/1
  Data Type Conversion/1 -> Product1/2
  Product1/1 -> Pulse/1
  Product/1 -> Relational Operator/2

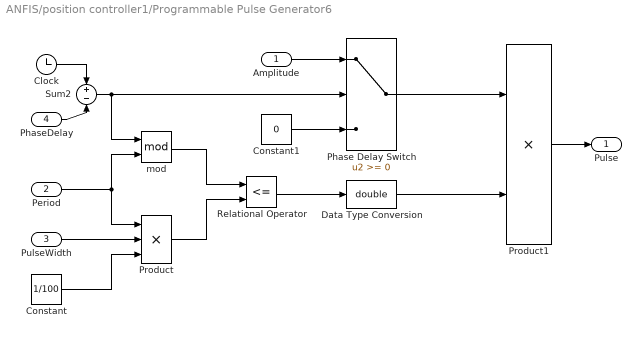
== system ANFIS/position controller1/Programmable Pulse Generator6 ==
  Amplitude : Inport
  Period : Inport  Port=2
  PulseWidth : Inport  Port=3
  PhaseDelay : Inport  Port=4
  Clock : Clock
  Constant : Constant  Value=1/100
  Constant1 : Constant  Value=0
  Data Type Conversion : DataTypeConversion  OutDataTypeStr=double
  Phase Delay Switch : Switch
  Product : Product  Inputs=3  RndMeth=Zero
  Product1 : Product  RndMeth=Zero
  Relational Operator : RelationalOperator  Operator=<=
  Sum2 : Sum  Inputs=+-
  mod : Math  Operator=mod  SaturateOnIntegerOverflow=on
  Pulse : Outport
  wires:
  Product/1 -> Relational Operator/2
  Product1/1 -> Pulse/1
  Data Type Conversion/1 -> Product1/2
  Relational Operator/1 -> Data Type Conversion/1
  Constant/1 -> Product/3
  PulseWidth/1 -> Product/2
  mod/1 -> Relational Operator/1
  Period/1 -> Product/1, mod/2
  Clock/1 -> Sum2/1
  PhaseDelay/1 -> Sum2/2
  Sum2/1 -> mod/1, Phase Delay Switch/2
  Amplitude/1 -> Phase Delay Switch/1
  Constant1/1 -> Phase Delay Switch/3
  Phase Delay Switch/1 -> Product1/1

== system ANFIS/position controller1/Programmable Pulse Generator7 ==
  Amplitude : Inport
  Period : Inport  Port=2
  PulseWidth : Inport  Port=3
  PhaseDelay : Inport  Port=4
  Clock : Clock
  Constant : Constant  Value=1/100
  Constant1 : Constant  Value=0
  Data Type Conversion : DataTypeConversion  OutDataTypeStr=double
  Phase Delay Switch : Switch
  Product : Product  Inputs=3  RndMeth=Zero
  Product1 : Product  RndMeth=Zero
  Relational Operator : RelationalOperator  Operator=<=
  Sum2 : Sum  Inputs=+-
  mod : Math  Operator=mod  SaturateOnIntegerOverflow=on
  Pulse : Outport
  wires:
  Phase Delay Switch/1 -> Product1/1
  Constant1/1 -> Phase Delay Switch/3
  Amplitude/1 -> Phase Delay Switch/1
  Sum2/1 -> Phase Delay Switch/2, mod/1
  PhaseDelay/1 -> Sum2/2
  Clock/1 -> Sum2/1
  Period/1 -> mod/2, Product/1
  mod/1 -> Relational Operator/1
  PulseWidth/1 -> Product/2
  Constant/1 -> Product/3
  Relational Operator/1 -> Data Type Conversion/1
  Data Type Conversion/1 -> Product1/2
  Product1/1 -> Pulse/1
  Product/1 -> Relational Operator/2

== system ANFIS/position controller1/Programmable Pulse Generator8 ==
  Amplitude : Inport
  Period : Inport  Port=2
  PulseWidth : Inport  Port=3
  PhaseDelay : Inport  Port=4
  Clock : Clock
  Constant : Constant  Value=1/100
  Constant1 : Constant  Value=0
  Data Type Conversion : DataTypeConversion  OutDataTypeStr=double
  Phase Delay Switch : Switch
  Product : Product  Inputs=3  RndMeth=Zero
  Product1 : Product  RndMeth=Zero
  Relational Operator : RelationalOperator  Operator=<=
  Sum2 : Sum  Inputs=+-
  mod : Math  Operator=mod  SaturateOnIntegerOverflow=on
  Pulse : Outport
  wires:
  Product/1 -> Relational Operator/2
  Product1/1 -> Pulse/1
  Data Type Conversion/1 -> Product1/2
  Relational Operator/1 -> Data Type Conversion/1
  Constant/1 -> Product/3
  PulseWidth/1 -> Product/2
  mod/1 -> Relational Operator/1
  Period/1 -> Product/1, mod/2
  Clock/1 -> Sum2/1
  PhaseDelay/1 -> Sum2/2
  Sum2/1 -> mod/1, Phase Delay Switch/2
  Amplitude/1 -> Phase Delay Switch/1
  Constant1/1 -> Phase Delay Switch/3
  Phase Delay Switch/1 -> Product1/1

== system ANFIS/position controller1/Programmable Pulse Generator9 ==
  Amplitude : Inport
  Period : Inport  Port=2
  PulseWidth : Inport  Port=3
  PhaseDelay : Inport  Port=4
  Clock : Clock
  Constant : Constant  Value=1/100
  Constant1 : Constant  Value=0
  Data Type Conversion : DataTypeConversion  OutDataTypeStr=double
  Phase Delay Switch : Switch
  Product : Product  Inputs=3  RndMeth=Zero
  Product1 : Product  RndMeth=Zero
  Relational Operator : RelationalOperator  Operator=<=
  Sum2 : Sum  Inputs=+-
  mod : Math  Operator=mod  SaturateOnIntegerOverflow=on
  Pulse : Outport
  wires:
  Phase Delay Switch/1 -> Product1/1
  Constant1/1 -> Phase Delay Switch/3
  Amplitude/1 -> Phase Delay Switch/1
  Sum2/1 -> Phase Delay Switch/2, mod/1
  PhaseDelay/1 -> Sum2/2
  Clock/1 -> Sum2/1
  Period/1 -> mod/2, Product/1
  mod/1 -> Relational Operator/1
  PulseWidth/1 -> Product/2
  Constant/1 -> Product/3
  Relational Operator/1 -> Data Type Conversion/1
  Data Type Conversion/1 -> Product1/2
  Product1/1 -> Pulse/1
  Product/1 -> Relational Operator/2

== system ANFIS/position controller2/Programmable Pulse Generator ==
  Amplitude : Inport
  Period : Inport  Port=2
  PulseWidth : Inport  Port=3
  PhaseDelay : Inport  Port=4
  Clock : Clock
  Constant : Constant  Value=1/100
  Constant1 : Constant  Value=0
  Data Type Conversion : DataTypeConversion  OutDataTypeStr=double
  Phase Delay Switch : Switch
  Product : Product  Inputs=3  RndMeth=Zero
  Product1 : Product  RndMeth=Zero
  Relational Operator : RelationalOperator  Operator=<=
  Sum2 : Sum  Inputs=+-
  mod : Math  Operator=mod  SaturateOnIntegerOverflow=on
  Pulse : Outport
  wires:
  Product/1 -> Relational Operator/2
  Product1/1 -> Pulse/1
  Data Type Conversion/1 -> Product1/2
  Relational Operator/1 -> Data Type Conversion/1
  Constant/1 -> Product/3
  PulseWidth/1 -> Product/2
  mod/1 -> Relational Operator/1
  Period/1 -> Product/1, mod/2
  Clock/1 -> Sum2/1
  PhaseDelay/1 -> Sum2/2
  Sum2/1 -> mod/1, Phase Delay Switch/2
  Amplitude/1 -> Phase Delay Switch/1
  Constant1/1 -> Phase Delay Switch/3
  Phase Delay Switch/1 -> Product1/1

== system ANFIS/position controller2/Programmable Pulse Generator1 ==
  Amplitude : Inport
  Period : Inport  Port=2
  PulseWidth : Inport  Port=3
  PhaseDelay : Inport  Port=4
  Clock : Clock
  Constant : Constant  Value=1/100
  Constant1 : Constant  Value=0
  Data Type Conversion : DataTypeConversion  OutDataTypeStr=double
  Phase Delay Switch : Switch
  Product : Product  Inputs=3  RndMeth=Zero
  Product1 : Product  RndMeth=Zero
  Relational Operator : RelationalOperator  Operator=<=
  Sum2 : Sum  Inputs=+-
  mod : Math  Operator=mod  SaturateOnIntegerOverflow=on
  Pulse : Outport
  wires:
  Phase Delay Switch/1 -> Product1/1
  Constant1/1 -> Phase Delay Switch/3
  Amplitude/1 -> Phase Delay Switch/1
  Sum2/1 -> Phase Delay Switch/2, mod/1
  PhaseDelay/1 -> Sum2/2
  Clock/1 -> Sum2/1
  Period/1 -> mod/2, Product/1
  mod/1 -> Relational Operator/1
  PulseWidth/1 -> Product/2
  Constant/1 -> Product/3
  Relational Operator/1 -> Data Type Conversion/1
  Data Type Conversion/1 -> Product1/2
  Product1/1 -> Pulse/1
  Product/1 -> Relational Operator/2

== system ANFIS/position controller2/Programmable Pulse Generator2 ==
  Amplitude : Inport
  Period : Inport  Port=2
  PulseWidth : Inport  Port=3
  PhaseDelay : Inport  Port=4
  Clock : Clock
  Constant : Constant  Value=1/100
  Constant1 : Constant  Value=0
  Data Type Conversion : DataTypeConversion  OutDataTypeStr=double
  Phase Delay Switch : Switch
  Product : Product  Inputs=3  RndMeth=Zero
  Product1 : Product  RndMeth=Zero
  Relational Operator : RelationalOperator  Operator=<=
  Sum2 : Sum  Inputs=+-
  mod : Math  Operator=mod  SaturateOnIntegerOverflow=on
  Pulse : Outport
  wires:
  Product/1 -> Relational Operator/2
  Product1/1 -> Pulse/1
  Data Type Conversion/1 -> Product1/2
  Relational Operator/1 -> Data Type Conversion/1
  Constant/1 -> Product/3
  PulseWidth/1 -> Product/2
  mod/1 -> Relational Operator/1
  Period/1 -> Product/1, mod/2
  Clock/1 -> Sum2/1
  PhaseDelay/1 -> Sum2/2
  Sum2/1 -> mod/1, Phase Delay Switch/2
  Amplitude/1 -> Phase Delay Switch/1
  Constant1/1 -> Phase Delay Switch/3
  Phase Delay Switch/1 -> Product1/1

== system ANFIS/position controller2/Programmable Pulse Generator3 ==
  Amplitude : Inport
  Period : Inport  Port=2
  PulseWidth : Inport  Port=3
  PhaseDelay : Inport  Port=4
  Clock : Clock
  Constant : Constant  Value=1/100
  Constant1 : Constant  Value=0
  Data Type Conversion : DataTypeConversion  OutDataTypeStr=double
  Phase Delay Switch : Switch
  Product : Product  Inputs=3  RndMeth=Zero
  Product1 : Product  RndMeth=Zero
  Relational Operator : RelationalOperator  Operator=<=
  Sum2 : Sum  Inputs=+-
  mod : Math  Operator=mod  SaturateOnIntegerOverflow=on
  Pulse : Outport
  wires:
  Phase Delay Switch/1 -> Product1/1
  Constant1/1 -> Phase Delay Switch/3
  Amplitude/1 -> Phase Delay Switch/1
  Sum2/1 -> Phase Delay Switch/2, mod/1
  PhaseDelay/1 -> Sum2/2
  Clock/1 -> Sum2/1
  Period/1 -> mod/2, Product/1
  mod/1 -> Relational Operator/1
  PulseWidth/1 -> Product/2
  Constant/1 -> Product/3
  Relational Operator/1 -> Data Type Conversion/1
  Data Type Conversion/1 -> Product1/2
  Product1/1 -> Pulse/1
  Product/1 -> Relational Operator/2

== system ANFIS/position controller2/Programmable Pulse Generator4 ==
  Amplitude : Inport
  Period : Inport  Port=2
  PulseWidth : Inport  Port=3
  PhaseDelay : Inport  Port=4
  Clock : Clock
  Constant : Constant  Value=1/100
  Constant1 : Constant  Value=0
  Data Type Conversion : DataTypeConversion  OutDataTypeStr=double
  Phase Delay Switch : Switch
  Product : Product  Inputs=3  RndMeth=Zero
  Product1 : Product  RndMeth=Zero
  Relational Operator : RelationalOperator  Operator=<=
  Sum2 : Sum  Inputs=+-
  mod : Math  Operator=mod  SaturateOnIntegerOverflow=on
  Pulse : Outport
  wires:
  Product/1 -> Relational Operator/2
  Product1/1 -> Pulse/1
  Data Type Conversion/1 -> Product1/2
  Relational Operator/1 -> Data Type Conversion/1
  Constant/1 -> Product/3
  PulseWidth/1 -> Product/2
  mod/1 -> Relational Operator/1
  Period/1 -> Product/1, mod/2
  Clock/1 -> Sum2/1
  PhaseDelay/1 -> Sum2/2
  Sum2/1 -> mod/1, Phase Delay Switch/2
  Amplitude/1 -> Phase Delay Switch/1
  Constant1/1 -> Phase Delay Switch/3
  Phase Delay Switch/1 -> Product1/1

== system ANFIS/position controller2/Programmable Pulse Generator5 ==
  Amplitude : Inport
  Period : Inport  Port=2
  PulseWidth : Inport  Port=3
  PhaseDelay : Inport  Port=4
  Clock : Clock
  Constant : Constant  Value=1/100
  Constant1 : Constant  Value=0
  Data Type Conversion : DataTypeConversion  OutDataTypeStr=double
  Phase Delay Switch : Switch
  Product : Product  Inputs=3  RndMeth=Zero
  Product1 : Product  RndMeth=Zero
  Relational Operator : RelationalOperator  Operator=<=
  Sum2 : Sum  Inputs=+-
  mod : Math  Operator=mod  SaturateOnIntegerOverflow=on
  Pulse : Outport
  wires:
  Phase Delay Switch/1 -> Product1/1
  Constant1/1 -> Phase Delay Switch/3
  Amplitude/1 -> Phase Delay Switch/1
  Sum2/1 -> Phase Delay Switch/2, mod/1
  PhaseDelay/1 -> Sum2/2
  Clock/1 -> Sum2/1
  Period/1 -> mod/2, Product/1
  mod/1 -> Relational Operator/1
  PulseWidth/1 -> Product/2
  Constant/1 -> Product/3
  Relational Operator/1 -> Data Type Conversion/1
  Data Type Conversion/1 -> Product1/2
  Product1/1 -> Pulse/1
  Product/1 -> Relational Operator/2

== system ANFIS/position controller2/Programmable Pulse Generator6 ==
  Amplitude : Inport
  Period : Inport  Port=2
  PulseWidth : Inport  Port=3
  PhaseDelay : Inport  Port=4
  Clock : Clock
  Constant : Constant  Value=1/100
  Constant1 : Constant  Value=0
  Data Type Conversion : DataTypeConversion  OutDataTypeStr=double
  Phase Delay Switch : Switch
  Product : Product  Inputs=3  RndMeth=Zero
  Product1 : Product  RndMeth=Zero
  Relational Operator : RelationalOperator  Operator=<=
  Sum2 : Sum  Inputs=+-
  mod : Math  Operator=mod  SaturateOnIntegerOverflow=on
  Pulse : Outport
  wires:
  Product/1 -> Relational Operator/2
  Product1/1 -> Pulse/1
  Data Type Conversion/1 -> Product1/2
  Relational Operator/1 -> Data Type Conversion/1
  Constant/1 -> Product/3
  PulseWidth/1 -> Product/2
  mod/1 -> Relational Operator/1
  Period/1 -> Product/1, mod/2
  Clock/1 -> Sum2/1
  PhaseDelay/1 -> Sum2/2
  Sum2/1 -> mod/1, Phase Delay Switch/2
  Amplitude/1 -> Phase Delay Switch/1
  Constant1/1 -> Phase Delay Switch/3
  Phase Delay Switch/1 -> Product1/1

== system ANFIS/position controller2/Programmable Pulse Generator7 ==
  Amplitude : Inport
  Period : Inport  Port=2
  PulseWidth : Inport  Port=3
  PhaseDelay : Inport  Port=4
  Clock : Clock
  Constant : Constant  Value=1/100
  Constant1 : Constant  Value=0
  Data Type Conversion : DataTypeConversion  OutDataTypeStr=double
  Phase Delay Switch : Switch
  Product : Product  Inputs=3  RndMeth=Zero
  Product1 : Product  RndMeth=Zero
  Relational Operator : RelationalOperator  Operator=<=
  Sum2 : Sum  Inputs=+-
  mod : Math  Operator=mod  SaturateOnIntegerOverflow=on
  Pulse : Outport
  wires:
  Phase Delay Switch/1 -> Product1/1
  Constant1/1 -> Phase Delay Switch/3
  Amplitude/1 -> Phase Delay Switch/1
  Sum2/1 -> Phase Delay Switch/2, mod/1
  PhaseDelay/1 -> Sum2/2
  Clock/1 -> Sum2/1
  Period/1 -> mod/2, Product/1
  mod/1 -> Relational Operator/1
  PulseWidth/1 -> Product/2
  Constant/1 -> Product/3
  Relational Operator/1 -> Data Type Conversion/1
  Data Type Conversion/1 -> Product1/2
  Product1/1 -> Pulse/1
  Product/1 -> Relational Operator/2

== system ANFIS/position controller2/Programmable Pulse Generator8 ==
  Amplitude : Inport
  Period : Inport  Port=2
  PulseWidth : Inport  Port=3
  PhaseDelay : Inport  Port=4
  Clock : Clock
  Constant : Constant  Value=1/100
  Constant1 : Constant  Value=0
  Data Type Conversion : DataTypeConversion  OutDataTypeStr=double
  Phase Delay Switch : Switch
  Product : Product  Inputs=3  RndMeth=Zero
  Product1 : Product  RndMeth=Zero
  Relational Operator : RelationalOperator  Operator=<=
  Sum2 : Sum  Inputs=+-
  mod : Math  Operator=mod  SaturateOnIntegerOverflow=on
  Pulse : Outport
  wires:
  Product/1 -> Relational Operator/2
  Product1/1 -> Pulse/1
  Data Type Conversion/1 -> Product1/2
  Relational Operator/1 -> Data Type Conversion/1
  Constant/1 -> Product/3
  PulseWidth/1 -> Product/2
  mod/1 -> Relational Operator/1
  Period/1 -> Product/1, mod/2
  Clock/1 -> Sum2/1
  PhaseDelay/1 -> Sum2/2
  Sum2/1 -> mod/1, Phase Delay Switch/2
  Amplitude/1 -> Phase Delay Switch/1
  Constant1/1 -> Phase Delay Switch/3
  Phase Delay Switch/1 -> Product1/1

== system ANFIS/position controller2/Programmable Pulse Generator9 ==
  Amplitude : Inport
  Period : Inport  Port=2
  PulseWidth : Inport  Port=3
  PhaseDelay : Inport  Port=4
  Clock : Clock
  Constant : Constant  Value=1/100
  Constant1 : Constant  Value=0
  Data Type Conversion : DataTypeConversion  OutDataTypeStr=double
  Phase Delay Switch : Switch
  Product : Product  Inputs=3  RndMeth=Zero
  Product1 : Product  RndMeth=Zero
  Relational Operator : RelationalOperator  Operator=<=
  Sum2 : Sum  Inputs=+-
  mod : Math  Operator=mod  SaturateOnIntegerOverflow=on
  Pulse : Outport
  wires:
  Phase Delay Switch/1 -> Product1/1
  Constant1/1 -> Phase Delay Switch/3
  Amplitude/1 -> Phase Delay Switch/1
  Sum2/1 -> Phase Delay Switch/2, mod/1
  PhaseDelay/1 -> Sum2/2
  Clock/1 -> Sum2/1
  Period/1 -> mod/2, Product/1
  mod/1 -> Relational Operator/1
  PulseWidth/1 -> Product/2
  Constant/1 -> Product/3
  Relational Operator/1 -> Data Type Conversion/1
  Data Type Conversion/1 -> Product1/2
  Product1/1 -> Pulse/1
  Product/1 -> Relational Operator/2

== system ANFIS/position controller3/Programmable Pulse Generator ==
  Amplitude : Inport
  Period : Inport  Port=2
  PulseWidth : Inport  Port=3
  PhaseDelay : Inport  Port=4
  Clock : Clock
  Constant : Constant  Value=1/100
  Constant1 : Constant  Value=0
  Data Type Conversion : DataTypeConversion  OutDataTypeStr=double
  Phase Delay Switch : Switch
  Product : Product  Inputs=3  RndMeth=Zero
  Product1 : Product  RndMeth=Zero
  Relational Operator : RelationalOperator  Operator=<=
  Sum2 : Sum  Inputs=+-
  mod : Math  Operator=mod  SaturateOnIntegerOverflow=on
  Pulse : Outport
  wires:
  Product/1 -> Relational Operator/2
  Product1/1 -> Pulse/1
  Data Type Conversion/1 -> Product1/2
  Relational Operator/1 -> Data Type Conversion/1
  Constant/1 -> Product/3
  PulseWidth/1 -> Product/2
  mod/1 -> Relational Operator/1
  Period/1 -> Product/1, mod/2
  Clock/1 -> Sum2/1
  PhaseDelay/1 -> Sum2/2
  Sum2/1 -> mod/1, Phase Delay Switch/2
  Amplitude/1 -> Phase Delay Switch/1
  Constant1/1 -> Phase Delay Switch/3
  Phase Delay Switch/1 -> Product1/1

== system ANFIS/position controller3/Programmable Pulse Generator1 ==
  Amplitude : Inport
  Period : Inport  Port=2
  PulseWidth : Inport  Port=3
  PhaseDelay : Inport  Port=4
  Clock : Clock
  Constant : Constant  Value=1/100
  Constant1 : Constant  Value=0
  Data Type Conversion : DataTypeConversion  OutDataTypeStr=double
  Phase Delay Switch : Switch
  Product : Product  Inputs=3  RndMeth=Zero
  Product1 : Product  RndMeth=Zero
  Relational Operator : RelationalOperator  Operator=<=
  Sum2 : Sum  Inputs=+-
  mod : Math  Operator=mod  SaturateOnIntegerOverflow=on
  Pulse : Outport
  wires:
  Phase Delay Switch/1 -> Product1/1
  Constant1/1 -> Phase Delay Switch/3
  Amplitude/1 -> Phase Delay Switch/1
  Sum2/1 -> Phase Delay Switch/2, mod/1
  PhaseDelay/1 -> Sum2/2
  Clock/1 -> Sum2/1
  Period/1 -> mod/2, Product/1
  mod/1 -> Relational Operator/1
  PulseWidth/1 -> Product/2
  Constant/1 -> Product/3
  Relational Operator/1 -> Data Type Conversion/1
  Data Type Conversion/1 -> Product1/2
  Product1/1 -> Pulse/1
  Product/1 -> Relational Operator/2
